simulink model "HydroPower"  (R2024b)
settings: Solver=ode4  StartTime=0.0  StopTime=200  FixedStep=0.001  RelTol=1e-3
values from neighbouring files (symbols this model uses):
  Af = 0.01    [Data__MOTOR.m]    (also in Generator_Data.m = 0.0001; Generator_Datatest.m)
  Bf = 0.0002    [Data__MOTOR.m]    (also in Generator_Data.m = 2e-05; Generator_Datatest.m)
  Cr = 0    [Generator_Data.m]
  CurrentFaultSwitch = 0    [Data__MOTOR.m]    (also in Generator_Data.m = 1; Generator_Datatest.m)
  f = 0.001    [Data__MOTOR.m]    (also in Generator_Data.m = 0)
  J = 0.0012    [Data__MOTOR.m]    (also in Generator_Data.m = 0.263; Generator_Datatest.m = 0.263)
  Ld = 1.4e-3+L_charge    (= 0.0014)    [Generator_Data.m]    (also in Generator_Datatest.m = 0.0231)
  Lq = 2.8e-3+L_charge    (= 0.0028)    [Generator_Data.m]    (also in Generator_Datatest.m = 0.0231)
  P = 4    [Generator_Data.m]    (also in Generator_Datatest.m = 3)
  Phif = 0.8    [Generator_Data.m]
  rate_noise_i = 0.02*In    (= 0.22)    [Data__MOTOR.m]    (also in Generator_Data.m = 0.02; Generator_Datatest.m)
  rate_noise_w = 0.02*Wn    (= 2.96)    [Data__MOTOR.m]    (also in Generator_Data.m = 0.002; Generator_Datatest.m)
  Rs = 0.6+R_charge    (= 0.6)    [Generator_Data.m]    (also in Generator_Datatest.m = 0.48)
  StartStop = 0    [Data__MOTOR.m]    (also in Generator_Data.m; Generator_Datatest.m)
  Te = 0.1    [Data__MOTOR.m]    (also in Generator_Data.m = 1; Generator_Datatest.m)
  Vd = 0    [Generator_Data.m]
  VelocityFaultSwitch = 0    [Data__MOTOR.m]    (also in Generator_Data.m = 1; Generator_Datatest.m)
  Vq = 0    [Generator_Data.m]
  wm = 2*pi*50/P    (= 78.5398163397)    [Generator_Data.m]
undefined symbols (not defined in the file or in its folder): dspblkCoreblockFVToolHelper, gcbh
libraries: SignalEditorBlockLib x3
(part 1 of 3)
settings Model: Creator=belka  LastModifiedBy=Nasser
settings DebuggingCC: SignalResolutionControl=TryResolveAll
settings RTWCC: GPUComputeCapability=3.5

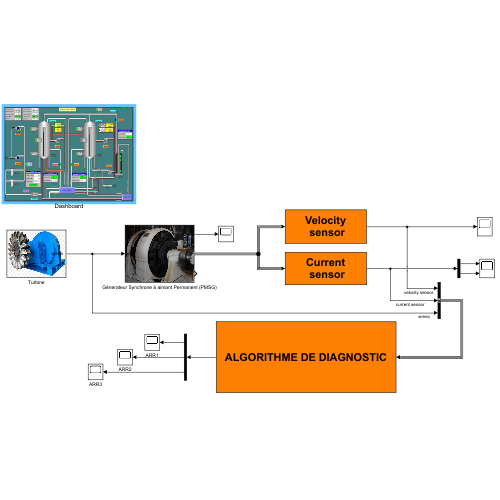
[thumbnail: Simulink's stored preview of the top-level diagram]
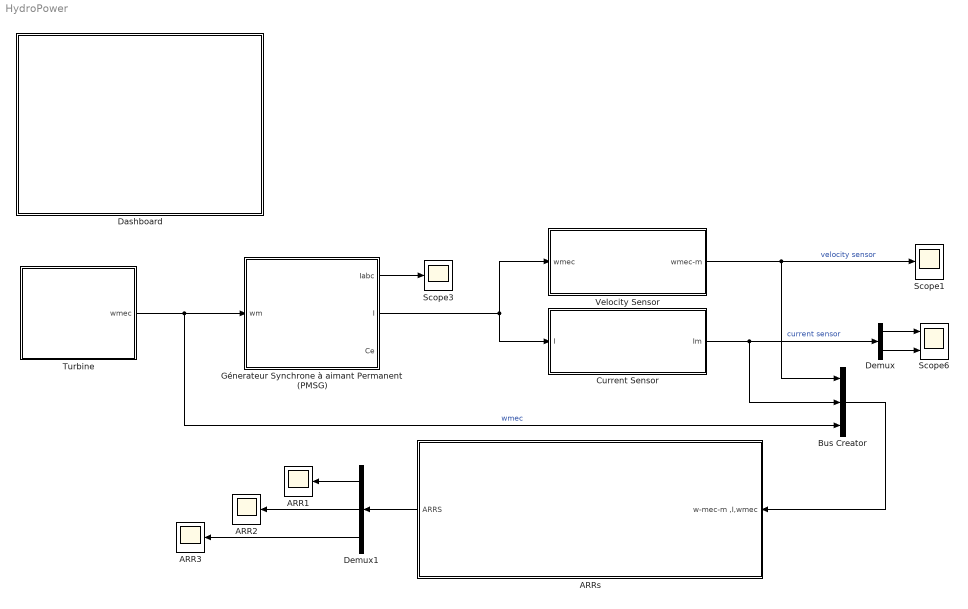
== system HydroPower ==
  ARR1 : Scope
  ARR2 : Scope
  ARR3 : Scope
  ARRs : Subsystem
      mask Display: disp('ALGORITHME DE DIAGNOSTIC')
  Bus Creator : BusCreator  Inputs=3
  Current Sensor : Subsystem
      mask Display: disp('Current\n sensor')
  Dashboard : Subsystem
      mask Display: image('scada.jpg');
  Demux : Demux  Outputs=2
  Demux1 : Demux  Outputs=3
  Génerateur Synchrone à aimant Permanent (PMSG) : Subsystem
      mask Display: image('generateur.png');
  Scope1 : Scope
  Scope3 : Scope
  Scope6 : Scope  NumInputPorts=2
  Turbine : Subsystem
      mask Display: image('turbine.png');
  Velocity Sensor : Subsystem
      mask Display: disp('Velocity\n sensor')
  wires:
  Turbine/1("wmec ") -> Bus Creator/3, Génerateur Synchrone à aimant Permanent (PMSG)/1("wm ")  "wmec"
  Génerateur Synchrone à aimant Permanent (PMSG)/1("Iabc ") -> Scope3/1
  Current Sensor/1(Im) -> Bus Creator/2, Demux/1  "current sensor"
  Demux/1 -> Scope6/1
  Demux/2 -> Scope6/2
  Bus Creator/1 -> ARRs/1(w-mec-m ,I,wmec)
  ARRs/1(ARRS) -> Demux1/1
  Demux1/1 -> ARR1/1
  Demux1/2 -> ARR2/1
  Demux1/3 -> ARR3/1
  Velocity Sensor/1(wmec-m) -> Bus Creator/1, Scope1/1  "velocity sensor"
  Génerateur Synchrone à aimant Permanent (PMSG)/2(I) -> Velocity Sensor/1(wmec), Current Sensor/1(I)

== system HydroPower/ARRs ==
  w-mec-m ,I,wmec : Inport
  ARR1 : Subsystem
      mask Display: disp('Residu 1')
  ARR2 : Subsystem
      mask Display: disp('Residu 2')
  ARR3 : Subsystem
      mask Display: disp('Residu 3')
  Bus Selector : BusSelector  OutputSignals=current sensor,velocity sensor
  Mux : Mux  Inputs=3
  ARRS : Outport  VectorParamsAs1DForOutWhenUnconnected=off
  wires:
  Bus Selector/1 -> ARR3/1(Id-m), ARR2/1(Id-m), ARR1/1(Id-m)  "<current sensor>"
  Bus Selector/2 -> ARR3/2(Wmec), ARR2/2(Wmec), ARR1/2(Wmec)  "<velocity sensor>"
  w-mec-m ,I,wmec/1 -> Bus Selector/1
  ARR1/1(R1) -> Mux/1
  ARR2/1(R1) -> Mux/2
  Mux/1 -> ARRS/1
  ARR3/1(R1) -> Mux/3

== system HydroPower/Current Sensor ==
  I : Inport
  Bus Selector : BusSelector  OutputSignals=Id,Iq
  Courrant Id : Subsystem
      mask Display:
      | color('black');
      | fprintf('Mesure\n Id','texmode','on');
      | 
      | %disp('Mesure\n I_{d}','texmode','on')
      | %color('yellow');
      | 
      | port_label('input', 1, 'I_{d}','texmode','on');
      | 
      | %color('green');
      | 
      | port_label('output', 1, 'I_{d-m}','texmode','on');
  Courrant Iq : Subsystem
      mask Display:
      | color('black');
      | fprintf('Mesure\n Iq','texmode','on');
      | 
      | %disp('Mesure\n I_{d}','texmode','on')
      | %color('yellow');
      | 
      | port_label('input', 1, 'I_{q}','texmode','on');
      | 
      | %color('green');
      | 
      | port_label('output', 1, 'I_{q-m}','texmode','on');
  Mux : Mux  Inputs=2
  Im : Outport  VectorParamsAs1DForOutWhenUnconnected=off
  wires:
  I/1 -> Bus Selector/1
  Bus Selector/1 -> Courrant Id/1(Id)  "<Id>"
  Courrant Id/1(Id-m) -> Mux/1
  Courrant Iq/1(Iq-m) -> Mux/2
  Mux/1 -> Im/1
  Bus Selector/2 -> Courrant Iq/1(In1)  "<Iq>"
